simulink model "MyTransmCU_RTW"  (Simulink 7.5)
settings: Solver=ode1  SolverMode=SingleTasking  StartTime=0.0  StopTime=inf  FixedStep=0.0002  RelTol=1e-3
PreLoadFcn:
  | vehicle = 'Car'; if ~length(which('cmcmd')), cmenv; end
  | MyTransmCU_RTW_bus
InitFcn:
  | vehicle = 'Car'; if ~length(which('cmcmd')), cmenv; end
  | MyTransmCU_RTW_bus
libraries: simulink x11
Description:
  | CarMaker Real-Time Target (generic)
settings Model: Creator=ml  LastModifiedBy=ml
settings DebuggingCC: SolverPrmCheckMsg=none
settings HardwareCC: TargetHWDeviceType=32-bit Generic  ProdEqTarget=off
settings RTWCC: SystemTargetFile=CarMaker.tlc  TemplateMakefile=CarMaker_unix.tmf  Description=CarMaker Real-Time Target (32-bit)  ProcessScript=CarMaker_make_rtw_hook
settings CodeAppCC: MaxIdLength=63
settings STFCustomTargetCC: ModelReferenceCompliant=off  GeneratePreprocessorConditionals=Disable all  SystemTargetFile=CarMaker.tlc
settings GRTTargetCC: ModelReferenceCompliant=off  ParMdlRefBuildCompliant=off  CompOptLevelCompliant=off  MatFileLogging=off  ExtModeMexFile=noextcomm
settings CustomProperty: DataType=string  Value=..
settings EnumStrPairs: String=Car

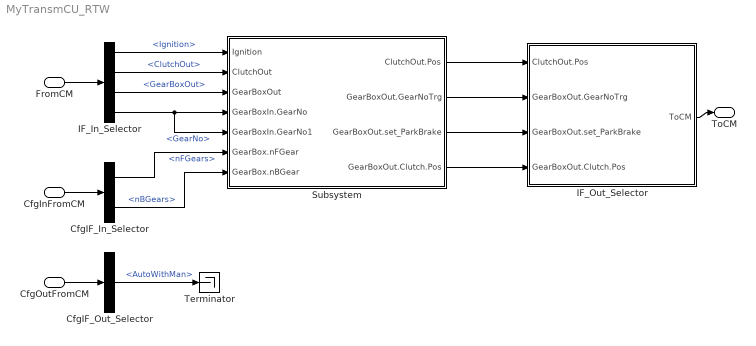
== system MyTransmCU_RTW ==
  FromCM : Inport  UseBusObject=on
      settings: BusObject=cmPTTransmCUIn
  CfgInFromCM : Inport  Port=2  UseBusObject=on
      settings: BusObject=cmPTTransmCUCfgIn
  CfgOutFromCM : Inport  Port=3  UseBusObject=on
      settings: BusObject=cmPTTransmCUCfgOut
  CfgIF_In_Selector : BusSelector  OutputSignals=GearBox.nFGears,GearBox.nBGears
  CfgIF_Out_Selector : BusSelector  OutputSignals=AutoWithMan
  IF_In_Selector : BusSelector  OutputSignals=Ignition,ClutchOut,GearBoxOut,GearBoxIn.GearNo
  IF_Out_Selector : Subsystem
      settings: OpenFcn=cmSignalSelect('SignalSelection_CB',gcb)
      mask Type: Signal Selection
      mask Description: Signal Selection Block
  Subsystem : Subsystem
  Terminator : Terminator
  ToCM : Outport  UseBusObject=on
      settings: BusObject=cmPTTransmCUOut
  wires:
  FromCM/1 -> IF_In_Selector/1
  IF_Out_Selector/1(ToCM) -> ToCM/1
  CfgInFromCM/1 -> CfgIF_In_Selector/1
  CfgOutFromCM/1 -> CfgIF_Out_Selector/1
  CfgIF_Out_Selector/1 -> Terminator/1  "<AutoWithMan>"
  IF_In_Selector/1 -> Subsystem/1(Ignition)  "<Ignition>"
  IF_In_Selector/2 -> Subsystem/2(ClutchOut)  "<ClutchOut>"
  IF_In_Selector/3 -> Subsystem/3(GearBoxOut)  "<GearBoxOut>"
  IF_In_Selector/4 -> Subsystem/4(GearBoxIn.GearNo), Subsystem/5(GearBoxIn.GearNo1)  "<GearNo>"
  Subsystem/1(ClutchOut.Pos) -> IF_Out_Selector/1(ClutchOut.Pos)
  Subsystem/2(GearBoxOut.GearNoTrg) -> IF_Out_Selector/2(GearBoxOut.GearNoTrg)
  Subsystem/3(GearBoxOut.set_ParkBrake) -> IF_Out_Selector/3(GearBoxOut.set_ParkBrake)
  Subsystem/4(GearBoxOut.Clutch.Pos) -> IF_Out_Selector/4(GearBoxOut.Clutch.Pos)
  CfgIF_In_Selector/1 -> Subsystem/6(GearBox.nFGear)  "<nFGears>"
  CfgIF_In_Selector/2 -> Subsystem/7(GearBox.nBGear)  "<nBGears>"

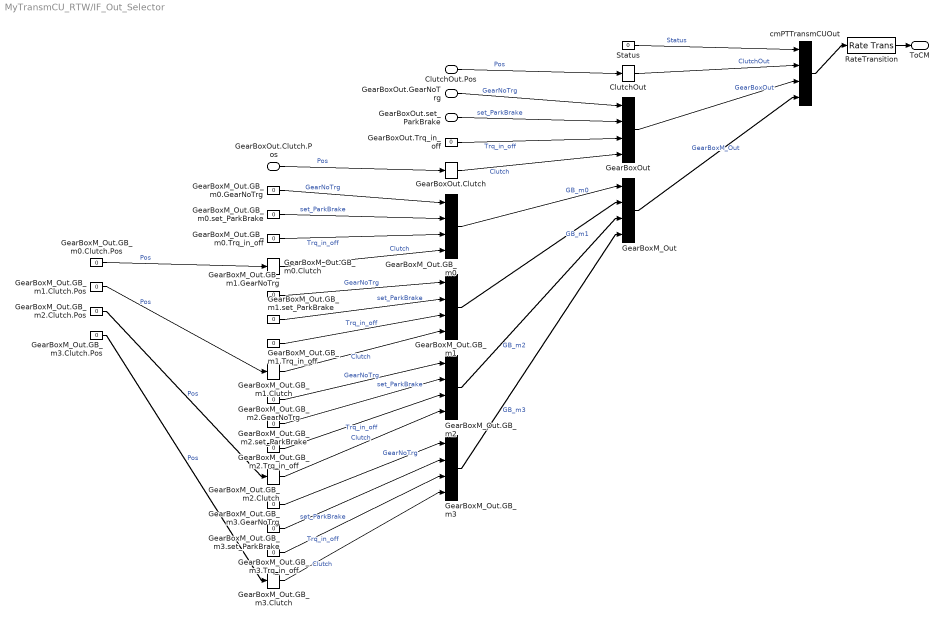
== system MyTransmCU_RTW/IF_Out_Selector ==
  ClutchOut.Pos : Inport
  GearBoxOut.GearNoTrg : Inport  Port=2
  GearBoxOut.set_ParkBrake : Inport  Port=3
  GearBoxOut.Clutch.Pos : Inport  Port=4
  ClutchOut : BusCreator  Inputs=1
  GearBoxM_Out : BusCreator
  GearBoxM_Out.GB_m{0..3} (4 alike) : BusCreator
  GearBoxM_Out.GB_m0.Clutch : BusCreator  Inputs=1
  GearBoxM_Out.GB_m0.Clutch.Pos : Constant  Value=0
  GearBoxM_Out.GB_m0.GearNoTrg : Constant  Value=0
  GearBoxM_Out.GB_m0.Trq_in_off : Constant  Value=0
  GearBoxM_Out.GB_m0.set_ParkBrake : Constant  Value=0
  GearBoxM_Out.GB_m1.Clutch : BusCreator  Inputs=1
  GearBoxM_Out.GB_m1.Clutch.Pos : Constant  Value=0
  GearBoxM_Out.GB_m1.GearNoTrg : Constant  Value=0
  GearBoxM_Out.GB_m1.Trq_in_off : Constant  Value=0
  GearBoxM_Out.GB_m1.set_ParkBrake : Constant  Value=0
  GearBoxM_Out.GB_m2.Clutch : BusCreator  Inputs=1
  GearBoxM_Out.GB_m2.Clutch.Pos : Constant  Value=0
  GearBoxM_Out.GB_m2.GearNoTrg : Constant  Value=0
  GearBoxM_Out.GB_m2.Trq_in_off : Constant  Value=0
  GearBoxM_Out.GB_m2.set_ParkBrake : Constant  Value=0
  GearBoxM_Out.GB_m3.Clutch : BusCreator  Inputs=1
  GearBoxM_Out.GB_m3.Clutch.Pos : Constant  Value=0
  GearBoxM_Out.GB_m3.GearNoTrg : Constant  Value=0
  GearBoxM_Out.GB_m3.Trq_in_off : Constant  Value=0
  GearBoxM_Out.GB_m3.set_ParkBrake : Constant  Value=0
  GearBoxOut : BusCreator
  GearBoxOut.Clutch : BusCreator  Inputs=1
  GearBoxOut.Trq_in_off : Constant  Value=0
  RateTransition : RateTransition  OutPortSampleTime=str2num(get_param(gcs,'FixedStep'))
  Status : Constant  Value=0
  cmPTTransmCUOut : BusCreator
  ToCM : Outport
  wires:
  RateTransition/1 -> ToCM/1
  cmPTTransmCUOut/1 -> RateTransition/1
  Status/1 -> cmPTTransmCUOut/1  "Status"
  ClutchOut/1 -> cmPTTransmCUOut/2  "ClutchOut"
  GearBoxOut/1 -> cmPTTransmCUOut/3  "GearBoxOut"
  GearBoxOut.Trq_in_off/1 -> GearBoxOut/3  "Trq_in_off"
  GearBoxOut.Clutch/1 -> GearBoxOut/4  "Clutch"
  GearBoxM_Out/1 -> cmPTTransmCUOut/4  "GearBoxM_Out"
  GearBoxM_Out.GB_m0/1 -> GearBoxM_Out/1  "GB_m0"
  GearBoxM_Out.GB_m0.GearNoTrg/1 -> GearBoxM_Out.GB_m0/1  "GearNoTrg"
  GearBoxM_Out.GB_m0.set_ParkBrake/1 -> GearBoxM_Out.GB_m0/2  "set_ParkBrake"
  GearBoxM_Out.GB_m0.Trq_in_off/1 -> GearBoxM_Out.GB_m0/3  "Trq_in_off"
  GearBoxM_Out.GB_m0.Clutch/1 -> GearBoxM_Out.GB_m0/4  "Clutch"
  GearBoxM_Out.GB_m0.Clutch.Pos/1 -> GearBoxM_Out.GB_m0.Clutch/1  "Pos"
  GearBoxM_Out.GB_m1/1 -> GearBoxM_Out/2  "GB_m1"
  GearBoxM_Out.GB_m1.GearNoTrg/1 -> GearBoxM_Out.GB_m1/1  "GearNoTrg"
  GearBoxM_Out.GB_m1.set_ParkBrake/1 -> GearBoxM_Out.GB_m1/2  "set_ParkBrake"
  GearBoxM_Out.GB_m1.Trq_in_off/1 -> GearBoxM_Out.GB_m1/3  "Trq_in_off"
  GearBoxM_Out.GB_m1.Clutch/1 -> GearBoxM_Out.GB_m1/4  "Clutch"
  GearBoxM_Out.GB_m1.Clutch.Pos/1 -> GearBoxM_Out.GB_m1.Clutch/1  "Pos"
  GearBoxM_Out.GB_m2/1 -> GearBoxM_Out/3  "GB_m2"
  GearBoxM_Out.GB_m2.GearNoTrg/1 -> GearBoxM_Out.GB_m2/1  "GearNoTrg"
  GearBoxM_Out.GB_m2.set_ParkBrake/1 -> GearBoxM_Out.GB_m2/2  "set_ParkBrake"
  GearBoxM_Out.GB_m2.Trq_in_off/1 -> GearBoxM_Out.GB_m2/3  "Trq_in_off"
  GearBoxM_Out.GB_m2.Clutch/1 -> GearBoxM_Out.GB_m2/4  "Clutch"
  GearBoxM_Out.GB_m2.Clutch.Pos/1 -> GearBoxM_Out.GB_m2.Clutch/1  "Pos"
  GearBoxM_Out.GB_m3/1 -> GearBoxM_Out/4  "GB_m3"
  GearBoxM_Out.GB_m3.GearNoTrg/1 -> GearBoxM_Out.GB_m3/1  "GearNoTrg"
  GearBoxM_Out.GB_m3.set_ParkBrake/1 -> GearBoxM_Out.GB_m3/2  "set_ParkBrake"
  GearBoxM_Out.GB_m3.Trq_in_off/1 -> GearBoxM_Out.GB_m3/3  "Trq_in_off"
  GearBoxM_Out.GB_m3.Clutch/1 -> GearBoxM_Out.GB_m3/4  "Clutch"
  GearBoxM_Out.GB_m3.Clutch.Pos/1 -> GearBoxM_Out.GB_m3.Clutch/1  "Pos"
  ClutchOut.Pos/1 -> ClutchOut/1  "Pos"
  GearBoxOut.GearNoTrg/1 -> GearBoxOut/1  "GearNoTrg"
  GearBoxOut.set_ParkBrake/1 -> GearBoxOut/2  "set_ParkBrake"
  GearBoxOut.Clutch.Pos/1 -> GearBoxOut.Clutch/1  "Pos"

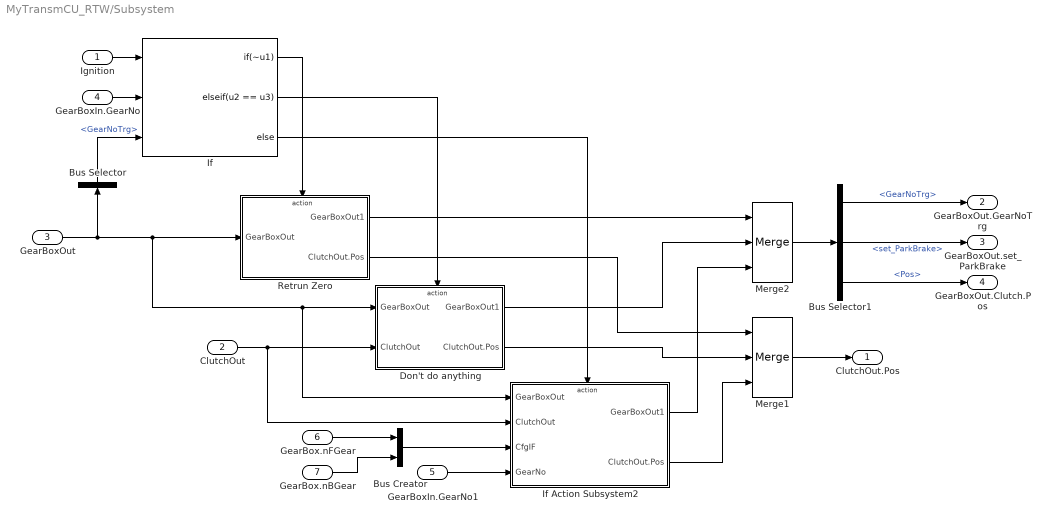
== system MyTransmCU_RTW/Subsystem ==
  Ignition : Inport  OutDataType=sfix(16)  OutScaling=2^0
  ClutchOut : Inport  Port=2  OutDataType=sfix(16)  OutScaling=2^0
  GearBoxOut : Inport  Port=3  OutDataType=sfix(16)  OutScaling=2^0
  GearBoxIn.GearNo : Inport  Port=4  OutDataType=sfix(16)  OutScaling=2^0
  GearBoxIn.GearNo1 : Inport  Port=5  OutDataType=sfix(16)  OutScaling=2^0
  GearBox.nFGear : Inport  Port=6  OutDataType=sfix(16)  OutScaling=2^0
  GearBox.nBGear : Inport  Port=7  OutDataType=sfix(16)  OutScaling=2^0
  Bus Creator : BusCreator  Inputs=2
  Bus Selector : BusSelector  OutputSignals=GearNoTrg
  Bus Selector1 : BusSelector  OutputSignals=GearNoTrg,set_ParkBrake,Clutch.Pos
  Don't do anything : Subsystem  TreatAsAtomicUnit=on
  If : If  NumInputs=3  IfExpression=~u1  ElseIfExpressions=u2 == u3
  If Action Subsystem2 : Subsystem  TreatAsAtomicUnit=on
  Merge1 : Merge  Inputs=3
  Merge2 : Merge  Inputs=3  InitialOutput=0
  Retrun Zero : Subsystem  TreatAsAtomicUnit=on
  ClutchOut.Pos : Outport  OutDataType=sfix(16)  OutScaling=2^0
  GearBoxOut.GearNoTrg : Outport  Port=2  OutDataType=sfix(16)  OutScaling=2^0
  GearBoxOut.set_ParkBrake : Outport  Port=3  OutDataType=sfix(16)  OutScaling=2^0
  GearBoxOut.Clutch.Pos : Outport  Port=4  OutDataType=sfix(16)  OutScaling=2^0
  wires:
  Ignition/1 -> If/1
  If/1 -> Retrun Zero/Action
  ClutchOut/1 -> Don't do anything/2(ClutchOut), If Action Subsystem2/2(ClutchOut)
  GearBoxOut/1 -> Bus Selector/1, Retrun Zero/1(GearBoxOut), Don't do anything/1(GearBoxOut), If Action Subsystem2/1(GearBoxOut)
  GearBoxIn.GearNo/1 -> If/2
  Bus Selector/1 -> If/3  "<GearNoTrg>"
  If/2 -> Don't do anything/Action
  If/3 -> If Action Subsystem2/Action
  GearBox.nFGear/1 -> Bus Creator/1
  GearBox.nBGear/1 -> Bus Creator/2
  Bus Creator/1 -> If Action Subsystem2/3(CfgIF)
  GearBoxIn.GearNo1/1 -> If Action Subsystem2/4(GearNo)
  Retrun Zero/2(ClutchOut.Pos) -> Merge1/1
  Don't do anything/2(ClutchOut.Pos) -> Merge1/2
  If Action Subsystem2/2(ClutchOut.Pos) -> Merge1/3
  Merge1/1 -> ClutchOut.Pos/1
  Retrun Zero/1(GearBoxOut1) -> Merge2/1
  Don't do anything/1(GearBoxOut1) -> Merge2/2
  If Action Subsystem2/1(GearBoxOut1) -> Merge2/3
  Merge2/1 -> Bus Selector1/1
  Bus Selector1/1 -> GearBoxOut.GearNoTrg/1  "<GearNoTrg>"
  Bus Selector1/2 -> GearBoxOut.set_ParkBrake/1  "<set_ParkBrake>"
  Bus Selector1/3 -> GearBoxOut.Clutch.Pos/1  "<Pos>"

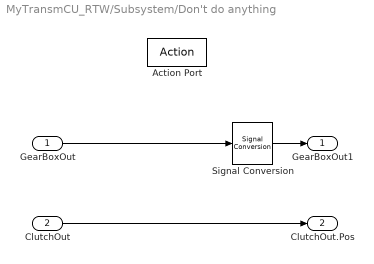
== system MyTransmCU_RTW/Subsystem/Don't do anything ==
  GearBoxOut : Inport  OutDataType=sfix(16)  OutScaling=2^0
  ClutchOut : Inport  Port=2  OutDataType=sfix(16)  OutScaling=2^0
  Action Port : ActionPort  ActionType=elseif
  Signal Conversion : SignalConversion  ConversionOutput=Bus copy
  GearBoxOut1 : Outport  OutDataType=sfix(16)  OutScaling=2^0
  ClutchOut.Pos : Outport  Port=2  OutDataType=sfix(16)  OutScaling=2^0
  wires:
  GearBoxOut/1 -> Signal Conversion/1
  ClutchOut/1 -> ClutchOut.Pos/1
  Signal Conversion/1 -> GearBoxOut1/1

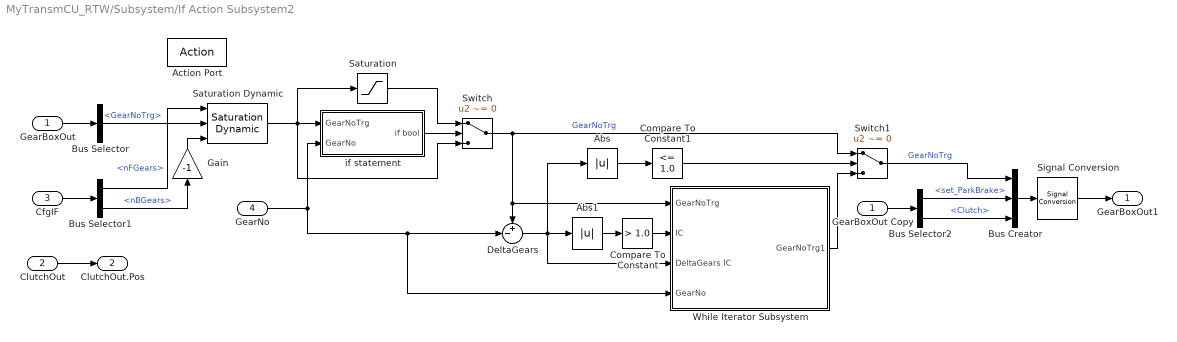
== system MyTransmCU_RTW/Subsystem/If Action Subsystem2 ==
  GearBoxOut : Inport  OutDataType=sfix(16)  OutScaling=2^0
  ClutchOut : Inport  Port=2  OutDataType=sfix(16)  OutScaling=2^0
  CfgIF : Inport  Port=3  OutDataType=sfix(16)  OutScaling=2^0
  GearNo : Inport  Port=4  OutDataType=sfix(16)  OutScaling=2^0
  Action Port : ActionPort  ActionType=else
  Abs : Abs  OutDataType=sfix(16)  OutScaling=2^0
  Abs1 : Abs  OutDataType=sfix(16)  OutScaling=2^0
  Bus Creator : BusCreator  Inputs=3
  Bus Selector : BusSelector  OutputSignals=GearNoTrg
  Bus Selector1 : BusSelector  OutputSignals=nFGears,nBGears
  Bus Selector2 : BusSelector  OutputSignals=set_ParkBrake,Clutch
  Compare To Constant : simulink/Logic and Bit Operations/Compare To Constant  SystemSampleTime=-1  relop=>  const=1.0  LogicOutDataTypeMode=uint8  ZeroCross=off
  Compare To Constant1 : simulink/Logic and Bit Operations/Compare To Constant  SystemSampleTime=-1  relop=<=  const=1.0  LogicOutDataTypeMode=uint8  ZeroCross=off
  DeltaGears : Sum  Inputs=+-|  OutDataType=sfix(16)  OutScaling=2^-10
  Gain : Gain  Gain=-1  ParameterDataType=sfix(16)  ParameterScaling=2^0  OutDataType=sfix(16)  OutScaling=2^0
  GearBoxOut Copy : InportShadow  Port=1  OutDataType=sfix(16)  OutScaling=2^0
  Saturation : Saturate  UpperLimit=1  LowerLimit=-1  OutDataType=sfix(16)  OutScaling=2^0
  Saturation Dynamic : simulink/Discontinuities/Saturation Dynamic  SystemSampleTime=-1  OutMin=[]  OutMax=[]  OutDataTypeStr=Inherit: Same as second input  OutDataType=sfix(16)  OutScaling=2^-10  DoSatur=off
  Signal Conversion : SignalConversion  ConversionOutput=Bus copy
  Switch : Switch  Criteria=u2 ~= 0  OutDataType=sfix(16)  OutScaling=2^0
  Switch1 : Switch  Criteria=u2 ~= 0  Threshold=1  OutDataType=sfix(16)  OutScaling=2^0
  While Iterator Subsystem : Subsystem  TreatAsAtomicUnit=on
  if statement : Subsystem
  GearBoxOut1 : Outport  OutDataType=sfix(16)  OutScaling=2^0
  ClutchOut.Pos : Outport  Port=2  OutDataType=sfix(16)  OutScaling=2^0
  wires:
  GearBoxOut/1 -> Bus Selector/1
  Bus Selector/1 -> Saturation Dynamic/2  "<GearNoTrg>"
  CfgIF/1 -> Bus Selector1/1
  Bus Selector1/1 -> Saturation Dynamic/1  "<nFGears>"
  Bus Selector1/2 -> Gain/1  "<nBGears>"
  Gain/1 -> Saturation Dynamic/3
  ClutchOut/1 -> ClutchOut.Pos/1
  GearNo/1 -> if statement/2(GearNo), DeltaGears/2, While Iterator Subsystem/4(GearNo)
  Saturation Dynamic/1 -> if statement/1(GearNoTrg), Switch/3, Saturation/1
  if statement/1(if bool) -> Switch/2
  Saturation/1 -> Switch/1
  Switch/1 -> While Iterator Subsystem/1(GearNoTrg), DeltaGears/1, Switch1/1  "GearNoTrg"
  DeltaGears/1 -> Abs/1, While Iterator Subsystem/3(DeltaGears IC), Abs1/1
  Abs/1 -> Compare To Constant1/1
  Bus Creator/1 -> Signal Conversion/1
  Abs1/1 -> Compare To Constant/1
  Compare To Constant/1 -> While Iterator Subsystem/2(IC)
  Bus Selector2/2 -> Bus Creator/3  "<Clutch>"
  Signal Conversion/1 -> GearBoxOut1/1
  Bus Selector2/1 -> Bus Creator/2  "<set_ParkBrake>"
  GearBoxOut Copy/1 -> Bus Selector2/1
  Compare To Constant1/1 -> Switch1/2
  While Iterator Subsystem/1(GearNoTrg1) -> Switch1/3
  Switch1/1 -> Bus Creator/1  "GearNoTrg"

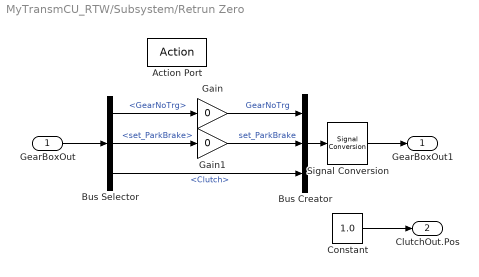
== system MyTransmCU_RTW/Subsystem/Retrun Zero ==
  GearBoxOut : Inport  OutDataType=sfix(16)  OutScaling=2^0
  Action Port : ActionPort  ActionType=then
  Bus Creator : BusCreator  Inputs=3
  Bus Selector : BusSelector  OutputSignals=GearNoTrg,set_ParkBrake,Clutch
  Constant : Constant  Value=1.0  OutDataType=sfix(16)  OutScaling=2^0
  Gain : Gain  Gain=0  ParameterDataType=sfix(16)  ParameterScaling=2^0  OutDataType=sfix(16)  OutScaling=2^0
  Gain1 : Gain  Gain=0  ParameterDataType=sfix(16)  ParameterScaling=2^0  OutDataType=sfix(16)  OutScaling=2^0
  Signal Conversion : SignalConversion  ConversionOutput=Bus copy
  GearBoxOut1 : Outport  OutDataType=sfix(16)  OutScaling=2^0
  ClutchOut.Pos : Outport  Port=2  OutDataType=sfix(16)  OutScaling=2^0  InitialOutput=1
  wires:
  Bus Selector/3 -> Bus Creator/3  "<Clutch>"
  Bus Selector/2 -> Gain1/1  "<set_ParkBrake>"
  Bus Selector/1 -> Gain/1  "<GearNoTrg>"
  Gain/1 -> Bus Creator/1  "GearNoTrg"
  Gain1/1 -> Bus Creator/2  "set_ParkBrake"
  GearBoxOut/1 -> Bus Selector/1
  Constant/1 -> ClutchOut.Pos/1
  Bus Creator/1 -> Signal Conversion/1
  Signal Conversion/1 -> GearBoxOut1/1

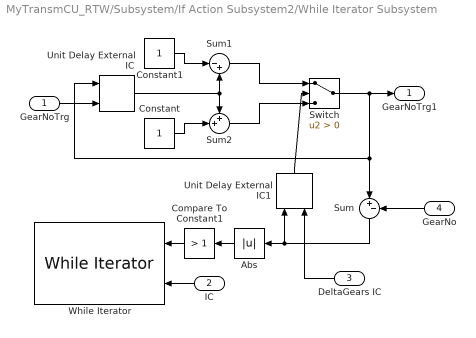
== system MyTransmCU_RTW/Subsystem/If Action Subsystem2/While Iterator Subsystem ==
  GearNoTrg : Inport  OutDataType=sfix(16)  OutScaling=2^0
  IC : Inport  Port=2  OutDataType=sfix(16)  OutScaling=2^0
  DeltaGears IC : Inport  Port=3  OutDataType=sfix(16)  OutScaling=2^0
  GearNo : Inport  Port=4  OutDataType=sfix(16)  OutScaling=2^0
  Abs : Abs  OutDataType=sfix(16)  OutScaling=2^0
  Compare To Constant1 : simulink/Logic and Bit Operations/Compare To Constant  SystemSampleTime=-1  relop=>  const=1  LogicOutDataTypeMode=uint8  ZeroCross=off
  Constant : Constant  OutDataType=sfix(16)  OutScaling=2^0
  Constant1 : Constant  OutDataType=sfix(16)  OutScaling=2^0
  Sum : Sum  Inputs=|+-  OutDataType=sfix(16)  OutScaling=2^0
  Sum1 : Sum  Inputs=|-+  OutDataType=sfix(16)  OutScaling=2^0
  Sum2 : Sum  Inputs=++|  OutDataType=sfix(16)  OutScaling=2^0
  Switch : Switch  Criteria=u2 > Threshold  OutDataType=sfix(16)  OutScaling=2^0
  Unit Delay External IC : simulink/Additional Math & Discrete/Additional Discrete/Unit Delay External IC  SystemSampleTime=-1  tsamp=-1
  Unit Delay External IC1 : simulink/Additional Math & Discrete/Additional Discrete/Unit Delay External IC  SystemSampleTime=-1  tsamp=-1
  While Iterator : WhileIterator  MaxIters=-1  ResetStates=reset
  GearNoTrg1 : Outport  OutDataType=sfix(16)  OutScaling=2^0
  wires:
  IC/1 -> While Iterator/2
  Switch/1 -> GearNoTrg1/1, Unit Delay External IC/1, Sum/1
  Sum/1 -> Abs/1, Unit Delay External IC1/1
  Sum1/1 -> Switch/1
  Sum2/1 -> Switch/3
  Constant/1 -> Sum2/2
  Constant1/1 -> Sum1/1
  Unit Delay External IC/1 -> Sum1/2, Sum2/1
  GearNoTrg/1 -> Unit Delay External IC/2
  Abs/1 -> Compare To Constant1/1
  Compare To Constant1/1 -> While Iterator/1
  Unit Delay External IC1/1 -> Switch/2
  GearNo/1 -> Sum/2
  DeltaGears IC/1 -> Unit Delay External IC1/2

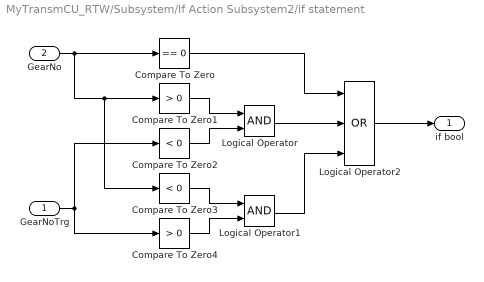
== system MyTransmCU_RTW/Subsystem/If Action Subsystem2/if statement ==
  GearNoTrg : Inport  OutDataType=sfix(16)  OutScaling=2^0
  GearNo : Inport  Port=2  OutDataType=sfix(16)  OutScaling=2^0
  Compare To Zero : simulink/Logic and Bit Operations/Compare To Zero  SystemSampleTime=-1  relop===  LogicOutDataTypeMode=uint8  ZeroCross=off
  Compare To Zero1 : simulink/Logic and Bit Operations/Compare To Zero  SystemSampleTime=-1  relop=>  LogicOutDataTypeMode=uint8  ZeroCross=off
  Compare To Zero2 : simulink/Logic and Bit Operations/Compare To Zero  SystemSampleTime=-1  relop=<  LogicOutDataTypeMode=uint8  ZeroCross=off
  Compare To Zero3 : simulink/Logic and Bit Operations/Compare To Zero  SystemSampleTime=-1  relop=<  LogicOutDataTypeMode=uint8  ZeroCross=off
  Compare To Zero4 : simulink/Logic and Bit Operations/Compare To Zero  SystemSampleTime=-1  relop=>  LogicOutDataTypeMode=uint8  ZeroCross=off
  Logical Operator : Logic  AllPortsSameDT=off  OutDataTypeMode=boolean  OutDataTypeStr=boolean
  Logical Operator1 : Logic  AllPortsSameDT=off  OutDataTypeMode=boolean  OutDataTypeStr=boolean
  Logical Operator2 : Logic  Operator=OR  Inputs=3  AllPortsSameDT=off  OutDataTypeMode=boolean  OutDataTypeStr=boolean
  if bool : Outport  OutDataType=sfix(16)  OutScaling=2^0
  wires:
  GearNo/1 -> Compare To Zero/1, Compare To Zero1/1, Compare To Zero3/1
  GearNoTrg/1 -> Compare To Zero2/1, Compare To Zero4/1
  Compare To Zero1/1 -> Logical Operator/1
  Compare To Zero2/1 -> Logical Operator/2
  Compare To Zero3/1 -> Logical Operator1/1
  Compare To Zero4/1 -> Logical Operator1/2
  Logical Operator2/1 -> if bool/1
  Compare To Zero/1 -> Logical Operator2/1
  Logical Operator/1 -> Logical Operator2/2
  Logical Operator1/1 -> Logical Operator2/3
